simulink model "single_step"  (R2024a)
settings: Solver=VariableStepAuto  StartTime=0.0  StopTime=10.0  RelTol=1e-3
settings Model: Creator=DNS  LastModifiedBy=DNS

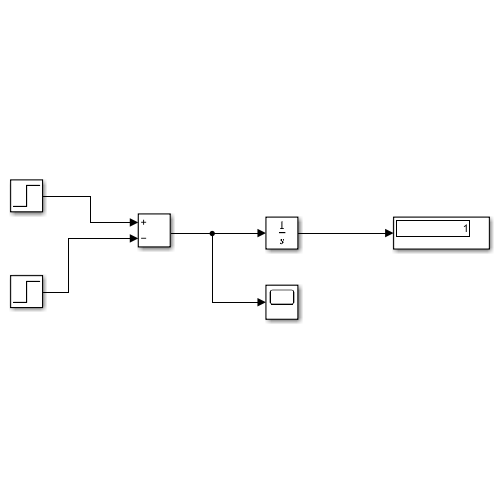
[thumbnail: Simulink's stored preview of the top-level diagram]
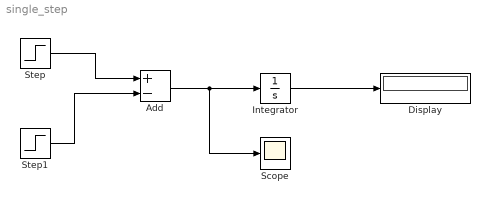
== system single_step ==
  Add : Sum  Inputs=+-
  Display : Display
  Integrator : Integrator
  Scope : Scope
  Step : Step  Time=0.5 - 0.005  After=100  SampleTime=0
  Step1 : Step  Time=0.5 + 0.005  After=100  SampleTime=0
  wires:
  Step/1 -> Add/1
  Step1/1 -> Add/2
  Add/1 -> Scope/1, Integrator/1
  Integrator/1 -> Display/1
